simulink library "ecrobot_nxt_lib"  (Simulink 6.4)
undefined symbols (not defined in the file or in its folder): BatteryVoltage, clearNXTSignalObjects, CompassSensorS1, EnterButton, GyroSensorS1, InitAccessorBlock, InitInterfaceBlock, LightSensorS1, RevolutionSensorA, RunButton, ServoMotorA, set_fcncallname, sfunxymap2, SoundSensorS1, SoundWAV, SystemClock, TouchSensorS1, TRACK_MAP, UltrasonicSensorS1
(part 2 of 2)

== system ecrobot_nxt_lib/JSP Semaphore ==
  System Outputs : Subsystem  mask(System Outputs){ShowInLibBrowser=0}
      mask prompts: ShowInLibBrowser "Mask Parameter 1:"
      mask help: Add code to a systems Outputs function
      settings: CopyFcn=%cccopyfcn(gcb)  OpenFcn=%ccopenfcn('System Outputs Function')
      mask Help: This block contains text fields to insert custom user code sections at the declaration, execution and exit sections of the systems outputs function.  By placing this block inside a subsytem, the custom user code will appear in that subsystems function.
      mask Display: disp('System\nOutputs');
  System Update : Subsystem  mask(System Update){ShowInLibBrowser=0}
      mask prompts: ShowInLibBrowser "Mask Parameter 1:"
      mask help: Add code to a systems Update function
      settings: CopyFcn=%cccopyfcn(gcb)  OpenFcn=%ccopenfcn('System Update Function')
      mask Help: This block contains text fields to insert custom user code sections at the declaration, execution and exit sections of the systems update function.  By placing this block inside a subsytem, the custom user code will appear in that subsystems function.
      mask Display: disp('System\nUpdate');

== system ecrobot_nxt_lib/Light Sensor Interface ==
  In1 : Inport
  Data Store Write : DataStoreWrite  DataStoreName=LightSensorS1  SampleTime=0.001
  Saturation : Saturate  UpperLimit=LightSensorS1.Max  LowerLimit=LightSensorS1.Min  SampleTime=0.001
  wires:
  In1/1 -> Saturation/1
  Saturation/1 -> Data Store Write/1

== system ecrobot_nxt_lib/Light Sensor Read ==
  Data Store Read : DataStoreRead  DataStoreName=LightSensorS1  SampleTime=-1
  Out1 : Outport
  wires:
  Data Store Read/1 -> Out1/1  "LightSensor_S1"

== system ecrobot_nxt_lib/NXT Color Sensor Interface ==
  In1 : Inport
  S-Function : S-Function  FunctionName=sfun_nxtcolor_sensor  Parameters=0.001,0,ip,bd_mode,sensor_mode
      mask init:
      | bd_mode = InitDeviceSFunBlock(bdroot);
  Saturation : Saturate  UpperLimit=1023  LowerLimit=0
  wires:
  Saturation/1 -> S-Function/1
  In1/1 -> Saturation/1

== system ecrobot_nxt_lib/OSEK Resource ==
  System Outputs : Subsystem  mask(System Outputs){ShowInLibBrowser=0}
      mask prompts: ShowInLibBrowser "Mask Parameter 1:"
      mask help: Add code to a systems Outputs function
      settings: CopyFcn=%cccopyfcn(gcb)  OpenFcn=%ccopenfcn('System Outputs Function')
      mask Help: This block contains text fields to insert custom user code sections at the declaration, execution and exit sections of the systems outputs function.  By placing this block inside a subsytem, the custom user code will appear in that subsystems function.
      mask Display: disp('System\nOutputs');
  System Update : Subsystem  mask(System Update){ShowInLibBrowser=0}
      mask prompts: ShowInLibBrowser "Mask Parameter 1:"
      mask help: Add code to a systems Update function
      settings: CopyFcn=%cccopyfcn(gcb)  OpenFcn=%ccopenfcn('System Update Function')
      mask Help: This block contains text fields to insert custom user code sections at the declaration, execution and exit sections of the systems update function.  By placing this block inside a subsytem, the custom user code will appear in that subsystems function.
      mask Display: disp('System\nUpdate');

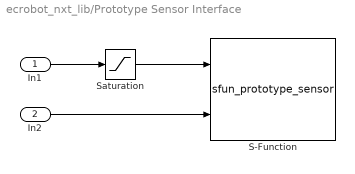
== system ecrobot_nxt_lib/Prototype Sensor Interface ==
  In1 : Inport
  In2 : Inport  Port=2
  S-Function : S-Function  FunctionName=sfun_prototype_sensor  Parameters=0.001,0,ip,bd_mode,4
      mask init:
      | bd_mode = InitDeviceSFunBlock(bdroot);
  Saturation : Saturate  UpperLimit=1023  LowerLimit=0
  wires:
  Saturation/1 -> S-Function/1
  In1/1 -> Saturation/1
  In2/1 -> S-Function/2

== system ecrobot_nxt_lib/Revolution Sensor Interface ==
  In1 : Inport
  Data Store Write : DataStoreWrite  DataStoreName=RevolutionSensorA  SampleTime=0.001
  Saturation : Saturate  UpperLimit=RevolutionSensorA.Max  LowerLimit=RevolutionSensorA.Min  SampleTime=0.001
  wires:
  In1/1 -> Saturation/1
  Saturation/1 -> Data Store Write/1

== system ecrobot_nxt_lib/Revolution Sensor Read ==
  Data Store Read : DataStoreRead  DataStoreName=RevolutionSensorA  SampleTime=-1
  Out1 : Outport
  wires:
  Data Store Read/1 -> Out1/1  "RevolutionSensor_A"

== system ecrobot_nxt_lib/Run Button Interface ==
  In1 : Inport
  Data Store Write : DataStoreWrite  DataStoreName=RunButton  SampleTime=0.001
  Saturation : Saturate  UpperLimit=RunButton.Max  LowerLimit=RunButton.Min  SampleTime=0.001
  wires:
  Saturation/1 -> Data Store Write/1
  In1/1 -> Saturation/1

== system ecrobot_nxt_lib/Run Button Read ==
  Data Store Read : DataStoreRead  DataStoreName=BatteryVoltage  SampleTime=-1
  Out1 : Outport
  wires:
  Data Store Read/1 -> Out1/1  "RunButton_"

== system ecrobot_nxt_lib/Servo Motor Interface ==
  Data Store Read : DataStoreRead  DataStoreName=ServoMotorA  SampleTime=0.001
  Saturation : Saturate  UpperLimit=ServoMotorA.Max  LowerLimit=ServoMotorA.Min  SampleTime=0.001
  Out1 : Outport
  wires:
  Data Store Read/1 -> Saturation/1
  Saturation/1 -> Out1/1

== system ecrobot_nxt_lib/Servo Motor Write ==
  In1 : Inport
  Data Store Write : DataStoreWrite  DataStoreName=ServoMotorA  SampleTime=-1
  wires:
  In1/1 -> Data Store Write/1

== system ecrobot_nxt_lib/Sound Sensor Interface ==
  In1 : Inport
  Data Store Write : DataStoreWrite  DataStoreName=SoundSensorS1  SampleTime=0.001
  Saturation : Saturate  UpperLimit=SoundSensorS1.Max  LowerLimit=SoundSensorS1.Min  SampleTime=0.001
  wires:
  In1/1 -> Saturation/1
  Saturation/1 -> Data Store Write/1

== system ecrobot_nxt_lib/Sound Sensor Read ==
  Data Store Read : DataStoreRead  DataStoreName=SoundSensorS1  SampleTime=-1
  Out1 : Outport
  wires:
  Data Store Read/1 -> Out1/1  "SoundSensor_S1"

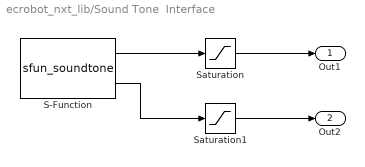
== system ecrobot_nxt_lib/Sound Tone  Interface ==
  S-Function : S-Function  FunctionName=sfun_soundtone  Parameters=0.001,0,bd_mode
      mask init:
      | bd_mode = InitDeviceSFunBlock(bdroot);
  Saturation : Saturate  UpperLimit=14080  LowerLimit=31
  Saturation1 : Saturate  UpperLimit=2560  LowerLimit=10
  Out1 : Outport
  Out2 : Outport  Port=2
  wires:
  S-Function/1 -> Saturation/1
  S-Function/2 -> Saturation1/1
  Saturation/1 -> Out1/1
  Saturation1/1 -> Out2/1

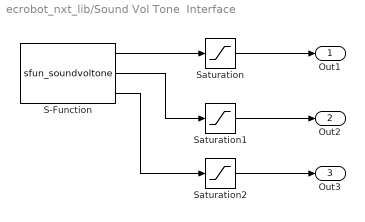
== system ecrobot_nxt_lib/Sound Vol Tone  Interface ==
  S-Function : S-Function  FunctionName=sfun_soundvoltone  Parameters=0.001,0,bd_mode
      mask init:
      | bd_mode = InitDeviceSFunBlock(bdroot);
  Saturation : Saturate  UpperLimit=14080  LowerLimit=31
  Saturation1 : Saturate  UpperLimit=2560  LowerLimit=10
  Saturation2 : Saturate  UpperLimit=100  LowerLimit=0
  Out1 : Outport
  Out2 : Outport  Port=2
  Out3 : Outport  Port=3
  wires:
  Saturation1/1 -> Out2/1
  Saturation/1 -> Out1/1
  S-Function/2 -> Saturation1/1
  S-Function/1 -> Saturation/1
  Saturation2/1 -> Out3/1
  S-Function/3 -> Saturation2/1

== system ecrobot_nxt_lib/Sound WAV Interface ==
  Data Store Read : DataStoreRead  DataStoreName=SoundWAV  SampleTime=0.001
  Saturation : Saturate  UpperLimit=SoundWAV.Max  LowerLimit=SoundWAV.Min  SampleTime=0.001
  Out1 : Outport
  wires:
  Saturation/1 -> Out1/1
  Data Store Read/1 -> Saturation/1

== system ecrobot_nxt_lib/Sound WAV Write ==
  In1 : Inport
  Data Store Write : DataStoreWrite  DataStoreName=SoundWAV  SampleTime=-1
  wires:
  In1/1 -> Data Store Write/1

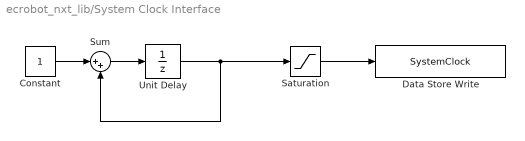
== system ecrobot_nxt_lib/System Clock Interface ==
  Constant : Constant  Value=1  OutDataTypeMode=uint32  OutDataType=sfix(16)  ConRadixGroup=Use specified scaling  OutScaling=2^0  SampleTime=inf  FramePeriod=inf
  Data Store Write : DataStoreWrite  DataStoreName=SystemClock  SampleTime=0.001
  Saturation : Saturate  UpperLimit=SystemClock.Max  LowerLimit=SystemClock.Min  SampleTime=0.001
  Sum : Sum  Inputs=|++  OutDataTypeMode=uint32
  Unit Delay : UnitDelay  SampleTime=0.001
  wires:
  Constant/1 -> Sum/1
  Sum/1 -> Unit Delay/1
  Saturation/1 -> Data Store Write/1
  Unit Delay/1 -> Saturation/1, Sum/2

== system ecrobot_nxt_lib/System Clock Read ==
  Data Store Read : DataStoreRead  DataStoreName=SystemClock  SampleTime=-1
  Out1 : Outport
  wires:
  Data Store Read/1 -> Out1/1  "SystemClock_"

== system ecrobot_nxt_lib/Touch Sensor Interface ==
  In1 : Inport
  Data Store Write : DataStoreWrite  DataStoreName=TouchSensorS1  SampleTime=0.001
  Saturation : Saturate  UpperLimit=TouchSensorS1.Max  LowerLimit=TouchSensorS1.Min  SampleTime=0.001
  wires:
  In1/1 -> Saturation/1
  Saturation/1 -> Data Store Write/1

== system ecrobot_nxt_lib/Touch Sensor Read ==
  Data Store Read : DataStoreRead  DataStoreName=TouchSensorS1  SampleTime=-1
  Out1 : Outport
  wires:
  Data Store Read/1 -> Out1/1  "TouchSensor_S1"

== system ecrobot_nxt_lib/USB Rx Interface ==
  In1 : Inport
  S-Function : S-Function  FunctionName=sfun_usb_rx  Parameters=0.001,0,bd_mode
      mask init:
      | bd_mode = InitDeviceSFunBlock(bdroot);
  Saturation : Saturate  UpperLimit=255  LowerLimit=0
  wires:
  In1/1 -> Saturation/1
  Saturation/1 -> S-Function/1

== system ecrobot_nxt_lib/USB Tx Interface ==
  S-Function : S-Function  FunctionName=sfun_usb_tx  Parameters=0.001,0,bd_mode
      mask init:
      | bd_mode = InitDeviceSFunBlock(bdroot);
  Saturation : Saturate  UpperLimit=255  LowerLimit=0
  Out1 : Outport
  wires:
  S-Function/1 -> Saturation/1
  Saturation/1 -> Out1/1

== system ecrobot_nxt_lib/Ultrasonic Sensor Interface ==
  In1 : Inport
  Data Store Write : DataStoreWrite  DataStoreName=UltrasonicSensorS1  SampleTime=0.001
  Saturation : Saturate  UpperLimit=UltrasonicSensorS1.Max  LowerLimit=UltrasonicSensorS1.Min  SampleTime=0.001
  wires:
  In1/1 -> Saturation/1
  Saturation/1 -> Data Store Write/1

== system ecrobot_nxt_lib/Ultrasonic Sensor Read ==
  Data Store Read : DataStoreRead  DataStoreName=UltrasonicSensorS1  SampleTime=-1
  Out1 : Outport
  wires:
  Data Store Read/1 -> Out1/1  "UltrasonicSensor_S1"

== system ecrobot_nxt_lib/Utilities for simulation ==
  XY Map Graph : Subsystem  LoadFcn=sfunxymap2([],[],[],'LoadBlock')  StartFcn=sfunxymap2([],[],[],'Start')  StopFcn=sfunxymap2([],[],[],'Stop')  TreatAsAtomicUnit=on  SimViewingDevice=on  mask(XYMAP scope.){xmin=0, xmax=200, ymin=0, ymax=200, map=TRACK_MAP}
      mask prompts: xmin "x-min:"; xmax "x-max:"; ymin "y-min:"; ymax "y-max:"; map "track map:"
      mask help: Plots second input (Y) against first input (X) at each time step to create an X-Y plot. Ignores data outside the ranges specified by x-min, x-max, y-min, y-max. bit map file (with '.bmp' extention) image is also plotted in the scope.
      settings: CopyFcn=sfunxymap2([],[],[],'CopyBlock')  DeleteFcn=sfunxymap2([],[],[],'DeleteBlock')  NameChangeFcn=sfunxymap2([],[],[],'NameChange')
      mask Help: This block can be used to explore limit cycles. Look at the m-file sfunxymap.m to see how it works.
      mask Display: plot([.05 .95 .95 .05 .05],[.45 .45 .95 .95 .45], 0.5+cos(0:0.1:2*pi)*0.3,0.7+sin(0:0.1:2*pi)*0.2)

== system ecrobot_nxt_lib/JSP Semaphore/System Outputs ==

== system ecrobot_nxt_lib/JSP Semaphore/System Update ==

== system ecrobot_nxt_lib/OSEK Resource/System Outputs ==

== system ecrobot_nxt_lib/OSEK Resource/System Update ==

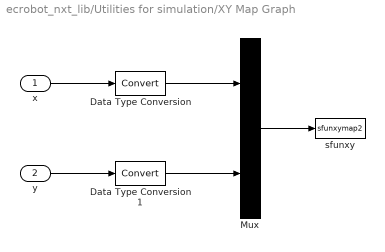
== system ecrobot_nxt_lib/Utilities for simulation/XY Map Graph ==
  x : Inport
  y : Inport  Port=2
  Data Type Conversion : DataTypeConversion  OutDataTypeMode=double
  Data Type Conversion1 : DataTypeConversion  OutDataTypeMode=double
  Mux : Mux  Inputs=2
  sfunxy : S-Function  FunctionName=sfunxymap2  Parameters=[xmin xmax ymin ymax], map
  wires:
  Mux/1 -> sfunxy/1
  x/1 -> Data Type Conversion/1
  y/1 -> Data Type Conversion1/1
  Data Type Conversion/1 -> Mux/1
  Data Type Conversion1/1 -> Mux/2
